simulink model "Scenario_3"  (R2020b)
settings: Solver=ode1  StartTime=0.0  StopTime=10.0  RelTol=1e-3
InitFcn:
  | Scenario_3_parameters;
values from neighbouring files (symbols this model uses):
  c0 = c0_zeb    (= 6.57988e-09)    [Scenario_17_parameters.m]    (also in Scenario_1_parameters.m = 6.37282e-09; Scenario_2_parameters.m = 6.37282e-09; Scenario_3_parameters.m)
  c0_hawk = 6.37282e-09    [Scenario_17_parameters.m]    (also in Scenario_1_parameters.m; Scenario_2_parameters.m; Scenario_3_parameters.m)
  c1 = c1_zeb    (= 9.15905e-09)    [Scenario_17_parameters.m]    (also in Scenario_1_parameters.m = 8.76156e-09; Scenario_2_parameters.m = 8.76156e-09; Scenario_3_parameters.m)
  c1_hawk = 8.76156e-09    [Scenario_17_parameters.m]    (also in Scenario_1_parameters.m; Scenario_2_parameters.m; Scenario_3_parameters.m)
  fg = 50    [Scenario_17_parameters.m]    (also in Scenario_1_parameters.m; Scenario_2_parameters.m; Scenario_3_parameters.m)
  G10gen = 0.85    [Scenario_3_parameters.m]
  G12gen = 0.85    [Scenario_3_parameters.m]
  G1gen = 0.50    (= 0.5)    [Scenario_17_parameters.m]    (also in Scenario_1_parameters.m = 0.2; Scenario_2_parameters.m = 0.1245; Scenario_3_parameters.m = 0.45)
  G2gen = 0.30    (= 0.3)    [Scenario_1_parameters.m]    (also in Scenario_2_parameters.m; Scenario_3_parameters.m = 0.4)
  G3gen = 0.25    [Scenario_1_parameters.m]    (also in Scenario_2_parameters.m = 0.2; Scenario_3_parameters.m = 0.6)
  G4gen = 0.95    [Scenario_3_parameters.m]
  G5gen = 0.75    [Scenario_17_parameters.m]    (also in Scenario_1_parameters.m = 0.22; Scenario_2_parameters.m = 0.2; Scenario_3_parameters.m = 0.7)
  G6gen = 0.90    (= 0.9)    [Scenario_17_parameters.m]    (also in Scenario_1_parameters.m = 0.41; Scenario_2_parameters.m = 0.2078; Scenario_3_parameters.m = 0.95)
  G7gen = 0.60    (= 0.6)    [Scenario_17_parameters.m]    (also in Scenario_1_parameters.m = 0.52; Scenario_2_parameters.m = 0.518; Scenario_3_parameters.m = 0.5)
  G8gen = 0.55    [Scenario_17_parameters.m]    (also in Scenario_3_parameters.m = 0.65)
  G9gen = 0.85    [Scenario_17_parameters.m]    (also in Scenario_3_parameters.m = 0.75)
  Ihvpk = Ihv*sqrt(2)    [Scenario_17_parameters.m]    (also in Scenario_1_parameters.m; Scenario_2_parameters.m; Scenario_3_parameters.m)
  l0 = l0_zeb    (= 0.00368)    [Scenario_17_parameters.m]    (also in Scenario_1_parameters.m = 0.00373; Scenario_2_parameters.m = 0.00373; Scenario_3_parameters.m)
  l0_hawk = 0.00373    [Scenario_17_parameters.m]    (also in Scenario_1_parameters.m; Scenario_2_parameters.m; Scenario_3_parameters.m)
  l1 = l1_zeb    (= 0.00128)    [Scenario_17_parameters.m]    (also in Scenario_1_parameters.m = 0.00133; Scenario_2_parameters.m = 0.00133; Scenario_3_parameters.m)
  L10dem = 0.10    (= 0.1)    [Scenario_3_parameters.m]
  L12dem = 0.025    [Scenario_17_parameters.m]    (also in Scenario_3_parameters.m = 0.005)
  L13dem = 0.005    [Scenario_3_parameters.m]
  l1_hawk = 0.00133    [Scenario_17_parameters.m]    (also in Scenario_1_parameters.m; Scenario_2_parameters.m; Scenario_3_parameters.m)
  L1dem = 0.25    [Scenario_17_parameters.m]    (also in Scenario_3_parameters.m = 0.1)
  L3dem = 0.30    (= 0.3)    [Scenario_17_parameters.m]    (also in Scenario_1_parameters.m = 0.1; Scenario_2_parameters.m = 0.1; Scenario_3_parameters.m = 0.2)
  L6dem = 0.15    [Scenario_1_parameters.m]    (also in Scenario_2_parameters.m; Scenario_3_parameters.m = 0.1)
  L7dem = 0.10    (= 0.1)    [Scenario_1_parameters.m]    (also in Scenario_2_parameters.m; Scenario_3_parameters.m = 0.15)
  L9dem = 0.15    [Scenario_17_parameters.m]    (also in Scenario_3_parameters.m)
  Pr = Sr*PF    (= 1900000000)    [Scenario_17_parameters.m]    (also in Scenario_1_parameters.m = 550050000; Scenario_2_parameters.m = 550050000; Scenario_3_parameters.m = 11640000000)
  Qr = sqrt(Sr^2 - Pr^2)    [Scenario_17_parameters.m]    (also in Scenario_1_parameters.m; Scenario_2_parameters.m; Scenario_3_parameters.m)
  r0 = r0_zeb    (= 0.39362)    [Scenario_17_parameters.m]    (also in Scenario_1_parameters.m = 0.44587; Scenario_2_parameters.m = 0.44587; Scenario_3_parameters.m)
  r0_hawk = 0.44587    [Scenario_17_parameters.m]    (also in Scenario_1_parameters.m; Scenario_2_parameters.m; Scenario_3_parameters.m)
  r1 = r1_zeb    (= 0.06862)    [Scenario_17_parameters.m]    (also in Scenario_1_parameters.m = 0.12087; Scenario_2_parameters.m = 0.12087; Scenario_3_parameters.m)
  r1_hawk = 0.12087    [Scenario_17_parameters.m]    (also in Scenario_1_parameters.m; Scenario_2_parameters.m; Scenario_3_parameters.m)
  Rtpu = Xtpu/40    (= 0.0025)    [Scenario_17_parameters.m]    (also in Scenario_1_parameters.m = 0.00375; Scenario_2_parameters.m = 0.00375; Scenario_3_parameters.m = 0.00375)
  S10non = 500e6    (= 500000000)    [Scenario_3_parameters.m]
  S12non = 1500e6    (= 1500000000)    [Scenario_3_parameters.m]
  S1non = 700e6    (= 700000000)    [Scenario_17_parameters.m]    (also in Scenario_1_parameters.m = 400000000; Scenario_2_parameters.m = 400000000; Scenario_3_parameters.m = 1000000000)
  S2non = 300e6    (= 300000000)    [Scenario_1_parameters.m]    (also in Scenario_2_parameters.m; Scenario_3_parameters.m = 3000000000)
  S3non = 200e6    (= 200000000)    [Scenario_1_parameters.m]    (also in Scenario_2_parameters.m; Scenario_3_parameters.m = 1000000000)
  S4non = 2000e6    (= 2000000000)    [Scenario_3_parameters.m]
  S5non = 400e6    (= 400000000)    [Scenario_17_parameters.m]    (also in Scenario_1_parameters.m = 500000000; Scenario_2_parameters.m = 500000000; Scenario_3_parameters.m = 2000000000)
  S6non = 150e6    (= 150000000)    [Scenario_17_parameters.m]    (also in Scenario_1_parameters.m = 400000000; Scenario_2_parameters.m = 400000000; Scenario_3_parameters.m = 3000000000)
  S7non = 1000e6    (= 1000000000)    [Scenario_17_parameters.m]    (also in Scenario_1_parameters.m = 200000000; Scenario_2_parameters.m = 200000000; Scenario_3_parameters.m = 4000000000)
  S8non = 600e6    (= 600000000)    [Scenario_17_parameters.m]    (also in Scenario_3_parameters.m = 2000000000)
  S9non = 200e6    (= 200000000)    [Scenario_17_parameters.m]    (also in Scenario_3_parameters.m = 1500000000)
  tonvsc = 0.01    [Scenario_17_parameters.m]    (also in Scenario_1_parameters.m = 0.02; Scenario_2_parameters.m; Scenario_3_parameters.m = 0.05)
  Ts = 100e-6    (= 0.0001)    [Scenario_17_parameters.m]    (also in Scenario_1_parameters.m; Scenario_2_parameters.m; Scenario_3_parameters.m = 5e-05)
  Vhv = 220e3    (= 220000)    [Scenario_17_parameters.m]    (also in Scenario_1_parameters.m; Scenario_2_parameters.m; Scenario_3_parameters.m)
  Vmv = 22e3    (= 22000)    [Scenario_17_parameters.m]    (also in Scenario_1_parameters.m; Scenario_2_parameters.m; Scenario_3_parameters.m)
  wc1 = wsw1/10    (= 848.230016469)    [Scenario_17_parameters.m]    (also in Scenario_1_parameters.m; Scenario_2_parameters.m; Scenario_3_parameters.m)
  wdc1 = wc1/10    (= 84.8230016469)    [Scenario_17_parameters.m]    (also in Scenario_1_parameters.m; Scenario_2_parameters.m; Scenario_3_parameters.m)
  wpq1 = wc1/10    (= 84.8230016469)    [Scenario_17_parameters.m]    (also in Scenario_1_parameters.m; Scenario_2_parameters.m; Scenario_3_parameters.m)
  wsw1 = ksw1*2*pi*fg    (= 8482.30016469)    [Scenario_17_parameters.m]    (also in Scenario_1_parameters.m; Scenario_2_parameters.m; Scenario_3_parameters.m)
  Xtpu = 0.10    (= 0.1)    [Scenario_17_parameters.m]    (also in Scenario_1_parameters.m = 0.15; Scenario_2_parameters.m = 0.15; Scenario_3_parameters.m = 0.15)
undefined symbols (not defined in the file or in its folder): D11, Delta, Kf, r, theta0
libraries: powerlib x426, simulink_extras x305, powerlib_meascontrol x139, pid_lib x109, eeGeneralControl x72, simulink x60, eeTransforms x54, spsFirstOrderFilterLib x36, eePwmGeneratorTwoLevel x9
(part 10 of 36)

== system Scenario_3/G4/VSC/VSC Model/EMT AVG ==
  Ref : Inport
  Controlled Voltage Source3 : powerlib/Electrical Sources/Controlled Voltage Source  Initialize=off  Source_Type=AC  Amplitude=Vhvpk  Phase=0  Frequency=fg  Measurements=None
  Controlled Voltage Source4 : powerlib/Electrical Sources/Controlled Voltage Source  Initialize=off  Source_Type=AC  Amplitude=Vhvpk  Phase=-2*pi/3  Frequency=fg  Measurements=None
  Controlled Voltage Source5 : powerlib/Electrical Sources/Controlled Voltage Source  Initialize=off  Source_Type=AC  Amplitude=Vhvpk  Phase=-4*pi/3  Frequency=fg  Measurements=None
  Demux1 : Demux  Outputs=3
  Ground : powerlib/Elements/Ground  LConnTagsString=a
  Ground4 : powerlib/Elements/Ground  LConnTagsString=a
  Ground5 : powerlib/Elements/Ground  LConnTagsString=a
  A : PMIOPort  Side=Left
  B : PMIOPort  Port=2  Side=Left
  C : PMIOPort  Port=3  Side=Left
  wires:
  Ref/1 -> Demux1/1
  Demux1/1 -> Controlled Voltage Source3/1
  Demux1/2 -> Controlled Voltage Source4/1
  Demux1/3 -> Controlled Voltage Source5/1
  connections:
  Controlled Voltage Source3/RConn1 -- A/RConn1
  Controlled Voltage Source4/RConn1 -- B/RConn1
  Controlled Voltage Source5/RConn1 -- C/RConn1
  Ground/LConn1 -- Controlled Voltage Source3/LConn1
  Ground4/LConn1 -- Controlled Voltage Source4/LConn1
  Ground5/LConn1 -- Controlled Voltage Source5/LConn1

== system Scenario_3/G4/VSC/VSC Model/EMT SW ==
  Ref : Inport
  DC Voltage Source : powerlib/Electrical Sources/DC Voltage Source  Amplitude=Vdc  Measurements=None
  Universal Bridge : powerlib/Power Electronics/Universal Bridge  Arms=3  SnubberResistance=1e6  SnubberCapacitance=inf  Device=IGBT / Diodes  Ron=1e-4  Lon=0  ForwardVoltages="[  0  0  ]"  ForwardVoltage=0  GTOparameters=[ 10e-6 , 20e-6 ]  IGBTparameters=[ 1e-6 , 2e-6 ]  Measurements=None  Measurements_2=None  converterType=Rectifier
  A : PMIOPort  Side=Left
  B : PMIOPort  Port=2  Side=Left
  C : PMIOPort  Port=3  Side=Left
  wires:
  Ref/1 -> Universal Bridge/1
  connections:
  Universal Bridge/LConn2 -- B/RConn1
  Universal Bridge/LConn1 -- A/RConn1
  Universal Bridge/LConn3 -- C/RConn1
  Universal Bridge/RConn1 -- DC Voltage Source/RConn1
  Universal Bridge/RConn2 -- DC Voltage Source/LConn1

== system Scenario_3/G4/VSC/VSC Model/Phasor ==
  Ref : Inport
  Controlled Current Source : powerlib/Electrical Sources/Controlled Current Source  Initialize=off  Source_Type=AC  Amplitude=0  Phase=0  Frequency=0  Measurements=None
  Controlled Current Source1 : powerlib/Electrical Sources/Controlled Current Source  Initialize=off  Source_Type=AC  Amplitude=0  Phase=0  Frequency=0  Measurements=None
  Controlled Current Source2 : powerlib/Electrical Sources/Controlled Current Source  Initialize=off  Source_Type=AC  Amplitude=0  Phase=0  Frequency=0  Measurements=None
  Demux1 : Demux  Outputs=3
  Ground{1..3,5} (4 alike) : powerlib/Elements/Ground  LConnTagsString=a
  Three-Phase Series RLC Branch : powerlib/Elements/Three-Phase Series RLC Branch  LConnTagsString=A|B|C  RConnTagsString=A|B|C  BranchType=R  Resistance=1e7  Inductance=1e-3  Capacitance=1e-6  Measurements=None
  A : PMIOPort  Side=Left
  B : PMIOPort  Port=2  Side=Left
  C : PMIOPort  Port=3  Side=Left
  wires:
  [c] -> Controlled Current Source2/1
  [b] -> Controlled Current Source1/1
  [a] -> Controlled Current Source/1
  Demux1/3 -> [c]
  Demux1/2 -> [b]
  Demux1/1 -> [a]
  Ref/1 -> Demux1/1
  connections:
  Controlled Current Source/RConn1 -- Ground1/LConn1
  Controlled Current Source1/RConn1 -- Ground2/LConn1
  Controlled Current Source2/RConn1 -- Ground3/LConn1
  A/RConn1 -- Controlled Current Source/LConn1 -- Three-Phase Series RLC Branch/LConn1
  C/RConn1 -- Controlled Current Source2/LConn1 -- Three-Phase Series RLC Branch/LConn3
  Ground5/LConn1 -- Three-Phase Series RLC Branch/RConn2 -- Three-Phase Series RLC Branch/RConn1 -- Three-Phase Series RLC Branch/RConn3
  Controlled Current Source1/LConn1 -- Three-Phase Series RLC Branch/LConn2 -- B/RConn1

== system Scenario_3/G6/VSC/VSC Control/Control loops ==
  note: 1) Add Subsystem or Model blocks as valid variant choices.
      | 2) You cannot connect blocks at this level. At simulation, connectivity is automatically
      | determined, based on the active variant and port name matching.
  Pset : Inport
  Qset : Inport  Port=2
  vqd+- : Inport  Port=3
  iqd+- : Inport  Port=4
  freq : Inport  Port=5
  Block : Inport  Port=6
  Phasor I 1st : Subsystem  VariantControl=Phasor_I_1st
  Phasor I ref : Subsystem  VariantControl=Phasor_I_ref
  Phasor PQ 1st : Subsystem  VariantControl=Phasor_PQ
  "SW, EMT AVG, Phasor Quasi-EMT" : Subsystem  VariantControl=EMT_and_QEMT
  vqd+-ref : Outport
  iqd+-ref : Outport  Port=2
  m : Outport  Port=3

== system Scenario_3/G6/VSC/VSC Control/Measurements ==
  note: 1) Add Subsystem or Model blocks as valid variant choices.
      | 2) You cannot connect blocks at this level. At simulation, connectivity is automatically
      | determined, based on the active variant and port name matching.
  Vabc : Inport
  Iabc : Inport  Port=2
  EMT : Subsystem  VariantControl=EMT
  Phasor : Subsystem  VariantControl=Phasor
  vqd+- : Outport
  iqd+- : Outport  Port=2
  freq : Outport  Port=3
  theta : Outport  Port=4
  PQabc : Outport  Port=5

== system Scenario_3/G6/VSC/VSC Control/Modulation ==
  note: 1) Add Subsystem or Model blocks as valid variant choices.
      | 2) You cannot connect blocks at this level. At simulation, connectivity is automatically
      | determined, based on the active variant and port name matching.
  vqd+- : Inport
  vqd+-* : Inport  Port=2
  iqd+-* : Inport  Port=3
  theta : Inport  Port=4
  EMT AVG : Subsystem  VariantControl=EMT_AVG
  EMT Switching : Subsystem  VariantControl=EMT_SW
  Phasor I and Phasor PQ : Subsystem  VariantControl=Phasor_I_and_PQ
  Phasor Quasi-EMT : Subsystem  VariantControl=Phasor_QEMT
  Ref : Outport

== system Scenario_3/G6/VSC/VSC Model/EMT AVG ==
  Ref : Inport
  Controlled Voltage Source3 : powerlib/Electrical Sources/Controlled Voltage Source  Initialize=off  Source_Type=AC  Amplitude=Vhvpk  Phase=0  Frequency=fg  Measurements=None
  Controlled Voltage Source4 : powerlib/Electrical Sources/Controlled Voltage Source  Initialize=off  Source_Type=AC  Amplitude=Vhvpk  Phase=-2*pi/3  Frequency=fg  Measurements=None
  Controlled Voltage Source5 : powerlib/Electrical Sources/Controlled Voltage Source  Initialize=off  Source_Type=AC  Amplitude=Vhvpk  Phase=-4*pi/3  Frequency=fg  Measurements=None
  Demux1 : Demux  Outputs=3
  Ground : powerlib/Elements/Ground  LConnTagsString=a
  Ground4 : powerlib/Elements/Ground  LConnTagsString=a
  Ground5 : powerlib/Elements/Ground  LConnTagsString=a
  A : PMIOPort  Side=Left
  B : PMIOPort  Port=2  Side=Left
  C : PMIOPort  Port=3  Side=Left
  wires:
  Ref/1 -> Demux1/1
  Demux1/1 -> Controlled Voltage Source3/1
  Demux1/2 -> Controlled Voltage Source4/1
  Demux1/3 -> Controlled Voltage Source5/1
  connections:
  Controlled Voltage Source3/RConn1 -- A/RConn1
  Controlled Voltage Source4/RConn1 -- B/RConn1
  Controlled Voltage Source5/RConn1 -- C/RConn1
  Ground/LConn1 -- Controlled Voltage Source3/LConn1
  Ground4/LConn1 -- Controlled Voltage Source4/LConn1
  Ground5/LConn1 -- Controlled Voltage Source5/LConn1

== system Scenario_3/G6/VSC/VSC Model/EMT SW ==
  Ref : Inport
  DC Voltage Source : powerlib/Electrical Sources/DC Voltage Source  Amplitude=Vdc  Measurements=None
  Universal Bridge : powerlib/Power Electronics/Universal Bridge  Arms=3  SnubberResistance=1e6  SnubberCapacitance=inf  Device=IGBT / Diodes  Ron=1e-4  Lon=0  ForwardVoltages="[  0  0  ]"  ForwardVoltage=0  GTOparameters=[ 10e-6 , 20e-6 ]  IGBTparameters=[ 1e-6 , 2e-6 ]  Measurements=None  Measurements_2=None  converterType=Rectifier
  A : PMIOPort  Side=Left
  B : PMIOPort  Port=2  Side=Left
  C : PMIOPort  Port=3  Side=Left
  wires:
  Ref/1 -> Universal Bridge/1
  connections:
  Universal Bridge/LConn2 -- B/RConn1
  Universal Bridge/LConn1 -- A/RConn1
  Universal Bridge/LConn3 -- C/RConn1
  Universal Bridge/RConn1 -- DC Voltage Source/RConn1
  Universal Bridge/RConn2 -- DC Voltage Source/LConn1

== system Scenario_3/G6/VSC/VSC Model/Phasor ==
  Ref : Inport
  Controlled Current Source : powerlib/Electrical Sources/Controlled Current Source  Initialize=off  Source_Type=AC  Amplitude=0  Phase=0  Frequency=0  Measurements=None
  Controlled Current Source1 : powerlib/Electrical Sources/Controlled Current Source  Initialize=off  Source_Type=AC  Amplitude=0  Phase=0  Frequency=0  Measurements=None
  Controlled Current Source2 : powerlib/Electrical Sources/Controlled Current Source  Initialize=off  Source_Type=AC  Amplitude=0  Phase=0  Frequency=0  Measurements=None
  Demux1 : Demux  Outputs=3
  Ground{1..3,5} (4 alike) : powerlib/Elements/Ground  LConnTagsString=a
  Three-Phase Series RLC Branch : powerlib/Elements/Three-Phase Series RLC Branch  LConnTagsString=A|B|C  RConnTagsString=A|B|C  BranchType=R  Resistance=1e7  Inductance=1e-3  Capacitance=1e-6  Measurements=None
  A : PMIOPort  Side=Left
  B : PMIOPort  Port=2  Side=Left
  C : PMIOPort  Port=3  Side=Left
  wires:
  [c] -> Controlled Current Source2/1
  [b] -> Controlled Current Source1/1
  [a] -> Controlled Current Source/1
  Demux1/3 -> [c]
  Demux1/2 -> [b]
  Demux1/1 -> [a]
  Ref/1 -> Demux1/1
  connections:
  Controlled Current Source/RConn1 -- Ground1/LConn1
  Controlled Current Source1/RConn1 -- Ground2/LConn1
  Controlled Current Source2/RConn1 -- Ground3/LConn1
  A/RConn1 -- Controlled Current Source/LConn1 -- Three-Phase Series RLC Branch/LConn1
  C/RConn1 -- Controlled Current Source2/LConn1 -- Three-Phase Series RLC Branch/LConn3
  Ground5/LConn1 -- Three-Phase Series RLC Branch/RConn2 -- Three-Phase Series RLC Branch/RConn1 -- Three-Phase Series RLC Branch/RConn3
  Controlled Current Source1/LConn1 -- Three-Phase Series RLC Branch/LConn2 -- B/RConn1

== system Scenario_3/G7/VSC/VSC Control/Control loops ==
  note: 1) Add Subsystem or Model blocks as valid variant choices.
      | 2) You cannot connect blocks at this level. At simulation, connectivity is automatically
      | determined, based on the active variant and port name matching.
  Pset : Inport
  Qset : Inport  Port=2
  vqd+- : Inport  Port=3
  iqd+- : Inport  Port=4
  freq : Inport  Port=5
  Block : Inport  Port=6
  Phasor I 1st : Subsystem  VariantControl=Phasor_I_1st
  Phasor I ref : Subsystem  VariantControl=Phasor_I_ref
  Phasor PQ 1st : Subsystem  VariantControl=Phasor_PQ
  "SW, EMT AVG, Phasor Quasi-EMT" : Subsystem  VariantControl=EMT_and_QEMT
  vqd+-ref : Outport
  iqd+-ref : Outport  Port=2
  m : Outport  Port=3

== system Scenario_3/G7/VSC/VSC Control/Measurements ==
  note: 1) Add Subsystem or Model blocks as valid variant choices.
      | 2) You cannot connect blocks at this level. At simulation, connectivity is automatically
      | determined, based on the active variant and port name matching.
  Vabc : Inport
  Iabc : Inport  Port=2
  EMT : Subsystem  VariantControl=EMT
  Phasor : Subsystem  VariantControl=Phasor
  vqd+- : Outport
  iqd+- : Outport  Port=2
  freq : Outport  Port=3
  theta : Outport  Port=4
  PQabc : Outport  Port=5

== system Scenario_3/G7/VSC/VSC Control/Modulation ==
  note: 1) Add Subsystem or Model blocks as valid variant choices.
      | 2) You cannot connect blocks at this level. At simulation, connectivity is automatically
      | determined, based on the active variant and port name matching.
  vqd+- : Inport
  vqd+-* : Inport  Port=2
  iqd+-* : Inport  Port=3
  theta : Inport  Port=4
  EMT AVG : Subsystem  VariantControl=EMT_AVG
  EMT Switching : Subsystem  VariantControl=EMT_SW
  Phasor I and Phasor PQ : Subsystem  VariantControl=Phasor_I_and_PQ
  Phasor Quasi-EMT : Subsystem  VariantControl=Phasor_QEMT
  Ref : Outport

== system Scenario_3/G7/VSC/VSC Model/EMT AVG ==
  Ref : Inport
  Controlled Voltage Source3 : powerlib/Electrical Sources/Controlled Voltage Source  Initialize=off  Source_Type=AC  Amplitude=Vhvpk  Phase=0  Frequency=fg  Measurements=None
  Controlled Voltage Source4 : powerlib/Electrical Sources/Controlled Voltage Source  Initialize=off  Source_Type=AC  Amplitude=Vhvpk  Phase=-2*pi/3  Frequency=fg  Measurements=None
  Controlled Voltage Source5 : powerlib/Electrical Sources/Controlled Voltage Source  Initialize=off  Source_Type=AC  Amplitude=Vhvpk  Phase=-4*pi/3  Frequency=fg  Measurements=None
  Demux1 : Demux  Outputs=3
  Ground : powerlib/Elements/Ground  LConnTagsString=a
  Ground4 : powerlib/Elements/Ground  LConnTagsString=a
  Ground5 : powerlib/Elements/Ground  LConnTagsString=a
  A : PMIOPort  Side=Left
  B : PMIOPort  Port=2  Side=Left
  C : PMIOPort  Port=3  Side=Left
  wires:
  Ref/1 -> Demux1/1
  Demux1/1 -> Controlled Voltage Source3/1
  Demux1/2 -> Controlled Voltage Source4/1
  Demux1/3 -> Controlled Voltage Source5/1
  connections:
  Controlled Voltage Source3/RConn1 -- A/RConn1
  Controlled Voltage Source4/RConn1 -- B/RConn1
  Controlled Voltage Source5/RConn1 -- C/RConn1
  Ground/LConn1 -- Controlled Voltage Source3/LConn1
  Ground4/LConn1 -- Controlled Voltage Source4/LConn1
  Ground5/LConn1 -- Controlled Voltage Source5/LConn1

== system Scenario_3/G7/VSC/VSC Model/EMT SW ==
  Ref : Inport
  DC Voltage Source : powerlib/Electrical Sources/DC Voltage Source  Amplitude=Vdc  Measurements=None
  Universal Bridge : powerlib/Power Electronics/Universal Bridge  Arms=3  SnubberResistance=1e6  SnubberCapacitance=inf  Device=IGBT / Diodes  Ron=1e-4  Lon=0  ForwardVoltages="[  0  0  ]"  ForwardVoltage=0  GTOparameters=[ 10e-6 , 20e-6 ]  IGBTparameters=[ 1e-6 , 2e-6 ]  Measurements=None  Measurements_2=None  converterType=Rectifier
  A : PMIOPort  Side=Left
  B : PMIOPort  Port=2  Side=Left
  C : PMIOPort  Port=3  Side=Left
  wires:
  Ref/1 -> Universal Bridge/1
  connections:
  Universal Bridge/LConn2 -- B/RConn1
  Universal Bridge/LConn1 -- A/RConn1
  Universal Bridge/LConn3 -- C/RConn1
  Universal Bridge/RConn1 -- DC Voltage Source/RConn1
  Universal Bridge/RConn2 -- DC Voltage Source/LConn1

== system Scenario_3/G7/VSC/VSC Model/Phasor ==
  Ref : Inport
  Controlled Current Source : powerlib/Electrical Sources/Controlled Current Source  Initialize=off  Source_Type=AC  Amplitude=0  Phase=0  Frequency=0  Measurements=None
  Controlled Current Source1 : powerlib/Electrical Sources/Controlled Current Source  Initialize=off  Source_Type=AC  Amplitude=0  Phase=0  Frequency=0  Measurements=None
  Controlled Current Source2 : powerlib/Electrical Sources/Controlled Current Source  Initialize=off  Source_Type=AC  Amplitude=0  Phase=0  Frequency=0  Measurements=None
  Demux1 : Demux  Outputs=3
  Ground{1..3,5} (4 alike) : powerlib/Elements/Ground  LConnTagsString=a
  Three-Phase Series RLC Branch : powerlib/Elements/Three-Phase Series RLC Branch  LConnTagsString=A|B|C  RConnTagsString=A|B|C  BranchType=R  Resistance=1e7  Inductance=1e-3  Capacitance=1e-6  Measurements=None
  A : PMIOPort  Side=Left
  B : PMIOPort  Port=2  Side=Left
  C : PMIOPort  Port=3  Side=Left
  wires:
  [c] -> Controlled Current Source2/1
  [b] -> Controlled Current Source1/1
  [a] -> Controlled Current Source/1
  Demux1/3 -> [c]
  Demux1/2 -> [b]
  Demux1/1 -> [a]
  Ref/1 -> Demux1/1
  connections:
  Controlled Current Source/RConn1 -- Ground1/LConn1
  Controlled Current Source1/RConn1 -- Ground2/LConn1
  Controlled Current Source2/RConn1 -- Ground3/LConn1
  A/RConn1 -- Controlled Current Source/LConn1 -- Three-Phase Series RLC Branch/LConn1
  C/RConn1 -- Controlled Current Source2/LConn1 -- Three-Phase Series RLC Branch/LConn3
  Ground5/LConn1 -- Three-Phase Series RLC Branch/RConn2 -- Three-Phase Series RLC Branch/RConn1 -- Three-Phase Series RLC Branch/RConn3
  Controlled Current Source1/LConn1 -- Three-Phase Series RLC Branch/LConn2 -- B/RConn1

== system Scenario_3/G9/VSC/VSC Control/Control loops ==
  note: 1) Add Subsystem or Model blocks as valid variant choices.
      | 2) You cannot connect blocks at this level. At simulation, connectivity is automatically
      | determined, based on the active variant and port name matching.
  Pset : Inport
  Qset : Inport  Port=2
  vqd+- : Inport  Port=3
  iqd+- : Inport  Port=4
  freq : Inport  Port=5
  Block : Inport  Port=6
  Phasor I 1st : Subsystem  VariantControl=Phasor_I_1st
  Phasor I ref : Subsystem  VariantControl=Phasor_I_ref
  Phasor PQ 1st : Subsystem  VariantControl=Phasor_PQ
  "SW, EMT AVG, Phasor Quasi-EMT" : Subsystem  VariantControl=EMT_and_QEMT
  vqd+-ref : Outport
  iqd+-ref : Outport  Port=2
  m : Outport  Port=3

== system Scenario_3/G9/VSC/VSC Control/Measurements ==
  note: 1) Add Subsystem or Model blocks as valid variant choices.
      | 2) You cannot connect blocks at this level. At simulation, connectivity is automatically
      | determined, based on the active variant and port name matching.
  Vabc : Inport
  Iabc : Inport  Port=2
  EMT : Subsystem  VariantControl=EMT
  Phasor : Subsystem  VariantControl=Phasor
  vqd+- : Outport
  iqd+- : Outport  Port=2
  freq : Outport  Port=3
  theta : Outport  Port=4
  PQabc : Outport  Port=5

== system Scenario_3/G9/VSC/VSC Control/Modulation ==
  note: 1) Add Subsystem or Model blocks as valid variant choices.
      | 2) You cannot connect blocks at this level. At simulation, connectivity is automatically
      | determined, based on the active variant and port name matching.
  vqd+- : Inport
  vqd+-* : Inport  Port=2
  iqd+-* : Inport  Port=3
  theta : Inport  Port=4
  EMT AVG : Subsystem  VariantControl=EMT_AVG
  EMT Switching : Subsystem  VariantControl=EMT_SW
  Phasor I and Phasor PQ : Subsystem  VariantControl=Phasor_I_and_PQ
  Phasor Quasi-EMT : Subsystem  VariantControl=Phasor_QEMT
  Ref : Outport

== system Scenario_3/G9/VSC/VSC Model/EMT AVG ==
  Ref : Inport
  Controlled Voltage Source3 : powerlib/Electrical Sources/Controlled Voltage Source  Initialize=off  Source_Type=AC  Amplitude=Vhvpk  Phase=0  Frequency=fg  Measurements=None
  Controlled Voltage Source4 : powerlib/Electrical Sources/Controlled Voltage Source  Initialize=off  Source_Type=AC  Amplitude=Vhvpk  Phase=-2*pi/3  Frequency=fg  Measurements=None
  Controlled Voltage Source5 : powerlib/Electrical Sources/Controlled Voltage Source  Initialize=off  Source_Type=AC  Amplitude=Vhvpk  Phase=-4*pi/3  Frequency=fg  Measurements=None
  Demux1 : Demux  Outputs=3
  Ground : powerlib/Elements/Ground  LConnTagsString=a
  Ground4 : powerlib/Elements/Ground  LConnTagsString=a
  Ground5 : powerlib/Elements/Ground  LConnTagsString=a
  A : PMIOPort  Side=Left
  B : PMIOPort  Port=2  Side=Left
  C : PMIOPort  Port=3  Side=Left
  wires:
  Ref/1 -> Demux1/1
  Demux1/1 -> Controlled Voltage Source3/1
  Demux1/2 -> Controlled Voltage Source4/1
  Demux1/3 -> Controlled Voltage Source5/1
  connections:
  Controlled Voltage Source3/RConn1 -- A/RConn1
  Controlled Voltage Source4/RConn1 -- B/RConn1
  Controlled Voltage Source5/RConn1 -- C/RConn1
  Ground/LConn1 -- Controlled Voltage Source3/LConn1
  Ground4/LConn1 -- Controlled Voltage Source4/LConn1
  Ground5/LConn1 -- Controlled Voltage Source5/LConn1

== system Scenario_3/G9/VSC/VSC Model/EMT SW ==
  Ref : Inport
  DC Voltage Source : powerlib/Electrical Sources/DC Voltage Source  Amplitude=Vdc  Measurements=None
  Universal Bridge : powerlib/Power Electronics/Universal Bridge  Arms=3  SnubberResistance=1e6  SnubberCapacitance=inf  Device=IGBT / Diodes  Ron=1e-4  Lon=0  ForwardVoltages="[  0  0  ]"  ForwardVoltage=0  GTOparameters=[ 10e-6 , 20e-6 ]  IGBTparameters=[ 1e-6 , 2e-6 ]  Measurements=None  Measurements_2=None  converterType=Rectifier
  A : PMIOPort  Side=Left
  B : PMIOPort  Port=2  Side=Left
  C : PMIOPort  Port=3  Side=Left
  wires:
  Ref/1 -> Universal Bridge/1
  connections:
  Universal Bridge/LConn2 -- B/RConn1
  Universal Bridge/LConn1 -- A/RConn1
  Universal Bridge/LConn3 -- C/RConn1
  Universal Bridge/RConn1 -- DC Voltage Source/RConn1
  Universal Bridge/RConn2 -- DC Voltage Source/LConn1

== system Scenario_3/G9/VSC/VSC Model/Phasor ==
  Ref : Inport
  Controlled Current Source : powerlib/Electrical Sources/Controlled Current Source  Initialize=off  Source_Type=AC  Amplitude=0  Phase=0  Frequency=0  Measurements=None
  Controlled Current Source1 : powerlib/Electrical Sources/Controlled Current Source  Initialize=off  Source_Type=AC  Amplitude=0  Phase=0  Frequency=0  Measurements=None
  Controlled Current Source2 : powerlib/Electrical Sources/Controlled Current Source  Initialize=off  Source_Type=AC  Amplitude=0  Phase=0  Frequency=0  Measurements=None
  Demux1 : Demux  Outputs=3
  Ground{1..3,5} (4 alike) : powerlib/Elements/Ground  LConnTagsString=a
  Three-Phase Series RLC Branch : powerlib/Elements/Three-Phase Series RLC Branch  LConnTagsString=A|B|C  RConnTagsString=A|B|C  BranchType=R  Resistance=1e7  Inductance=1e-3  Capacitance=1e-6  Measurements=None
  A : PMIOPort  Side=Left
  B : PMIOPort  Port=2  Side=Left
  C : PMIOPort  Port=3  Side=Left
  wires:
  [c] -> Controlled Current Source2/1
  [b] -> Controlled Current Source1/1
  [a] -> Controlled Current Source/1
  Demux1/3 -> [c]
  Demux1/2 -> [b]
  Demux1/1 -> [a]
  Ref/1 -> Demux1/1
  connections:
  Controlled Current Source/RConn1 -- Ground1/LConn1
  Controlled Current Source1/RConn1 -- Ground2/LConn1
  Controlled Current Source2/RConn1 -- Ground3/LConn1
  A/RConn1 -- Controlled Current Source/LConn1 -- Three-Phase Series RLC Branch/LConn1
  C/RConn1 -- Controlled Current Source2/LConn1 -- Three-Phase Series RLC Branch/LConn3
  Ground5/LConn1 -- Three-Phase Series RLC Branch/RConn2 -- Three-Phase Series RLC Branch/RConn1 -- Three-Phase Series RLC Branch/RConn3
  Controlled Current Source1/LConn1 -- Three-Phase Series RLC Branch/LConn2 -- B/RConn1

== system Scenario_3/HVDC interconnection/VSC1/VSC Control/Control loops ==
  note: 1) Add Subsystem or Model blocks as valid variant choices.
      | 2) You cannot connect blocks at this level. At simulation, connectivity is automatically
      | determined, based on the active variant and port name matching.
  Pset : Inport
  Qset : Inport  Port=2
  vqd+- : Inport  Port=3
  iqd+- : Inport  Port=4
  freq : Inport  Port=5
  Block : Inport  Port=6
  Phasor I 1st : Subsystem  VariantControl=Phasor_I_1st
  Phasor I ref : Subsystem  VariantControl=Phasor_I_ref
  Phasor PQ 1st : Subsystem  VariantControl=Phasor_PQ
  "SW, EMT AVG, Phasor Quasi-EMT" : Subsystem  VariantControl=EMT_and_QEMT
  vqd+-ref : Outport
  iqd+-ref : Outport  Port=2
  m : Outport  Port=3

== system Scenario_3/HVDC interconnection/VSC1/VSC Control/Measurements ==
  note: 1) Add Subsystem or Model blocks as valid variant choices.
      | 2) You cannot connect blocks at this level. At simulation, connectivity is automatically
      | determined, based on the active variant and port name matching.
  Vabc : Inport
  Iabc : Inport  Port=2
  EMT : Subsystem  VariantControl=EMT
  Phasor : Subsystem  VariantControl=Phasor
  vqd+- : Outport
  iqd+- : Outport  Port=2
  freq : Outport  Port=3
  theta : Outport  Port=4
  PQabc : Outport  Port=5

== system Scenario_3/HVDC interconnection/VSC1/VSC Control/Modulation ==
  note: 1) Add Subsystem or Model blocks as valid variant choices.
      | 2) You cannot connect blocks at this level. At simulation, connectivity is automatically
      | determined, based on the active variant and port name matching.
  vqd+- : Inport
  vqd+-* : Inport  Port=2
  iqd+-* : Inport  Port=3
  theta : Inport  Port=4
  EMT AVG : Subsystem  VariantControl=EMT_AVG
  EMT Switching : Subsystem  VariantControl=EMT_SW
  Phasor I and Phasor PQ : Subsystem  VariantControl=Phasor_I_and_PQ
  Phasor Quasi-EMT : Subsystem  VariantControl=Phasor_QEMT
  Ref : Outport

== system Scenario_3/HVDC interconnection/VSC1/VSC Model/EMT AVG ==
  Ref : Inport
  Controlled Voltage Source3 : powerlib/Electrical Sources/Controlled Voltage Source  Initialize=off  Source_Type=AC  Amplitude=Vhvpk  Phase=0  Frequency=fg  Measurements=None
  Controlled Voltage Source4 : powerlib/Electrical Sources/Controlled Voltage Source  Initialize=off  Source_Type=AC  Amplitude=Vhvpk  Phase=-2*pi/3  Frequency=fg  Measurements=None
  Controlled Voltage Source5 : powerlib/Electrical Sources/Controlled Voltage Source  Initialize=off  Source_Type=AC  Amplitude=Vhvpk  Phase=-4*pi/3  Frequency=fg  Measurements=None
  Demux1 : Demux  Outputs=3
  Ground : powerlib/Elements/Ground  LConnTagsString=a
  Ground4 : powerlib/Elements/Ground  LConnTagsString=a
  Ground5 : powerlib/Elements/Ground  LConnTagsString=a
  A : PMIOPort  Side=Left
  B : PMIOPort  Port=2  Side=Left
  C : PMIOPort  Port=3  Side=Left
  wires:
  Ref/1 -> Demux1/1
  Demux1/1 -> Controlled Voltage Source3/1
  Demux1/2 -> Controlled Voltage Source4/1
  Demux1/3 -> Controlled Voltage Source5/1
  connections:
  Controlled Voltage Source3/RConn1 -- A/RConn1
  Controlled Voltage Source4/RConn1 -- B/RConn1
  Controlled Voltage Source5/RConn1 -- C/RConn1
  Ground/LConn1 -- Controlled Voltage Source3/LConn1
  Ground4/LConn1 -- Controlled Voltage Source4/LConn1
  Ground5/LConn1 -- Controlled Voltage Source5/LConn1

== system Scenario_3/HVDC interconnection/VSC1/VSC Model/EMT SW ==
  Ref : Inport
  DC Voltage Source : powerlib/Electrical Sources/DC Voltage Source  Amplitude=Vdc  Measurements=None
  Universal Bridge : powerlib/Power Electronics/Universal Bridge  Arms=3  SnubberResistance=1e6  SnubberCapacitance=inf  Device=IGBT / Diodes  Ron=1e-4  Lon=0  ForwardVoltages="[  0  0  ]"  ForwardVoltage=0  GTOparameters=[ 10e-6 , 20e-6 ]  IGBTparameters=[ 1e-6 , 2e-6 ]  Measurements=None  Measurements_2=None  converterType=Rectifier
  A : PMIOPort  Side=Left
  B : PMIOPort  Port=2  Side=Left
  C : PMIOPort  Port=3  Side=Left
  wires:
  Ref/1 -> Universal Bridge/1
  connections:
  Universal Bridge/LConn2 -- B/RConn1
  Universal Bridge/LConn1 -- A/RConn1
  Universal Bridge/LConn3 -- C/RConn1
  Universal Bridge/RConn1 -- DC Voltage Source/RConn1
  Universal Bridge/RConn2 -- DC Voltage Source/LConn1

== system Scenario_3/HVDC interconnection/VSC1/VSC Model/Phasor ==
  Ref : Inport
  Controlled Current Source : powerlib/Electrical Sources/Controlled Current Source  Initialize=off  Source_Type=AC  Amplitude=0  Phase=0  Frequency=0  Measurements=None
  Controlled Current Source1 : powerlib/Electrical Sources/Controlled Current Source  Initialize=off  Source_Type=AC  Amplitude=0  Phase=0  Frequency=0  Measurements=None
  Controlled Current Source2 : powerlib/Electrical Sources/Controlled Current Source  Initialize=off  Source_Type=AC  Amplitude=0  Phase=0  Frequency=0  Measurements=None
  Demux1 : Demux  Outputs=3
  Ground{1..3,5} (4 alike) : powerlib/Elements/Ground  LConnTagsString=a
  Three-Phase Series RLC Branch : powerlib/Elements/Three-Phase Series RLC Branch  LConnTagsString=A|B|C  RConnTagsString=A|B|C  BranchType=R  Resistance=1e7  Inductance=1e-3  Capacitance=1e-6  Measurements=None
  A : PMIOPort  Side=Left
  B : PMIOPort  Port=2  Side=Left
  C : PMIOPort  Port=3  Side=Left
  wires:
  [c] -> Controlled Current Source2/1
  [b] -> Controlled Current Source1/1
  [a] -> Controlled Current Source/1
  Demux1/3 -> [c]
  Demux1/2 -> [b]
  Demux1/1 -> [a]
  Ref/1 -> Demux1/1
  connections:
  Controlled Current Source/RConn1 -- Ground1/LConn1
  Controlled Current Source1/RConn1 -- Ground2/LConn1
  Controlled Current Source2/RConn1 -- Ground3/LConn1
  A/RConn1 -- Controlled Current Source/LConn1 -- Three-Phase Series RLC Branch/LConn1
  C/RConn1 -- Controlled Current Source2/LConn1 -- Three-Phase Series RLC Branch/LConn3
  Ground5/LConn1 -- Three-Phase Series RLC Branch/RConn2 -- Three-Phase Series RLC Branch/RConn1 -- Three-Phase Series RLC Branch/RConn3
  Controlled Current Source1/LConn1 -- Three-Phase Series RLC Branch/LConn2 -- B/RConn1

== system Scenario_3/HVDC interconnection/VSC2/VSC Control/Control loops ==
  note: 1) Add Subsystem or Model blocks as valid variant choices.
      | 2) You cannot connect blocks at this level. At simulation, connectivity is automatically
      | determined, based on the active variant and port name matching.
  Pset : Inport
  Qset : Inport  Port=2
  vqd+- : Inport  Port=3
  iqd+- : Inport  Port=4
  freq : Inport  Port=5
  Block : Inport  Port=6
  Edc : Inport  Port=7
  Phasor I 1st : Subsystem  VariantControl=Phasor_I_1st
  Phasor I ref : Subsystem  VariantControl=Phasor_I_ref
  Phasor PQ 1st : Subsystem  VariantControl=Phasor_PQ
  "SW, EMT AVG, Phasor Quasi-EMT" : Subsystem  VariantControl=EMT_and_QEMT
  vqd+-ref : Outport
  iqd+-ref : Outport  Port=2
  m : Outport  Port=3

== system Scenario_3/HVDC interconnection/VSC2/VSC Control/Measurements ==
  note: 1) Add Subsystem or Model blocks as valid variant choices.
      | 2) You cannot connect blocks at this level. At simulation, connectivity is automatically
      | determined, based on the active variant and port name matching.
  Vabc : Inport
  Iabc : Inport  Port=2
  EMT : Subsystem  VariantControl=EMT
  Phasor : Subsystem  VariantControl=Phasor
  vqd+- : Outport
  iqd+- : Outport  Port=2
  freq : Outport  Port=3
  theta : Outport  Port=4
  PQabc : Outport  Port=5

== system Scenario_3/HVDC interconnection/VSC2/VSC Control/Modulation ==
  note: 1) Add Subsystem or Model blocks as valid variant choices.
      | 2) You cannot connect blocks at this level. At simulation, connectivity is automatically
      | determined, based on the active variant and port name matching.
  vqd+- : Inport
  vqd+-* : Inport  Port=2
  iqd+-* : Inport  Port=3
  theta : Inport  Port=4
  EMT AVG : Subsystem  VariantControl=EMT_AVG
  EMT Switching : Subsystem  VariantControl=EMT_SW
  Phasor I and Phasor PQ : Subsystem  VariantControl=Phasor_I_and_PQ
  Phasor Quasi-EMT : Subsystem  VariantControl=Phasor_QEMT
  Ref : Outport

== system Scenario_3/HVDC interconnection/VSC2/VSC Model/EMT AVG ==
  Ref : Inport
  Controlled Voltage Source3 : powerlib/Electrical Sources/Controlled Voltage Source  Initialize=off  Source_Type=AC  Amplitude=Vhvpk  Phase=0  Frequency=fg  Measurements=None
  Controlled Voltage Source4 : powerlib/Electrical Sources/Controlled Voltage Source  Initialize=off  Source_Type=AC  Amplitude=Vhvpk  Phase=-2*pi/3  Frequency=fg  Measurements=None
  Controlled Voltage Source5 : powerlib/Electrical Sources/Controlled Voltage Source  Initialize=off  Source_Type=AC  Amplitude=Vhvpk  Phase=-4*pi/3  Frequency=fg  Measurements=None
  Demux1 : Demux  Outputs=3
  Ground : powerlib/Elements/Ground  LConnTagsString=a
  Ground4 : powerlib/Elements/Ground  LConnTagsString=a
  Ground5 : powerlib/Elements/Ground  LConnTagsString=a
  A : PMIOPort  Side=Left
  B : PMIOPort  Port=2  Side=Left
  C : PMIOPort  Port=3  Side=Left
  wires:
  Ref/1 -> Demux1/1
  Demux1/1 -> Controlled Voltage Source3/1
  Demux1/2 -> Controlled Voltage Source4/1
  Demux1/3 -> Controlled Voltage Source5/1
  connections:
  Controlled Voltage Source3/RConn1 -- A/RConn1
  Controlled Voltage Source4/RConn1 -- B/RConn1
  Controlled Voltage Source5/RConn1 -- C/RConn1
  Ground/LConn1 -- Controlled Voltage Source3/LConn1
  Ground4/LConn1 -- Controlled Voltage Source4/LConn1
  Ground5/LConn1 -- Controlled Voltage Source5/LConn1

== system Scenario_3/HVDC interconnection/VSC2/VSC Model/EMT SW ==
  Ref : Inport
  DC Voltage Source : powerlib/Electrical Sources/DC Voltage Source  Amplitude=Vdc  Measurements=None
  Universal Bridge : powerlib/Power Electronics/Universal Bridge  Arms=3  SnubberResistance=1e6  SnubberCapacitance=inf  Device=IGBT / Diodes  Ron=1e-4  Lon=0  ForwardVoltages="[  0  0  ]"  ForwardVoltage=0  GTOparameters=[ 10e-6 , 20e-6 ]  IGBTparameters=[ 1e-6 , 2e-6 ]  Measurements=None  Measurements_2=None  converterType=Rectifier
  A : PMIOPort  Side=Left
  B : PMIOPort  Port=2  Side=Left
  C : PMIOPort  Port=3  Side=Left
  wires:
  Ref/1 -> Universal Bridge/1
  connections:
  Universal Bridge/LConn2 -- B/RConn1
  Universal Bridge/LConn1 -- A/RConn1
  Universal Bridge/LConn3 -- C/RConn1
  Universal Bridge/RConn1 -- DC Voltage Source/RConn1
  Universal Bridge/RConn2 -- DC Voltage Source/LConn1

== system Scenario_3/HVDC interconnection/VSC2/VSC Model/Phasor ==
  Ref : Inport
  Controlled Current Source : powerlib/Electrical Sources/Controlled Current Source  Initialize=off  Source_Type=AC  Amplitude=0  Phase=0  Frequency=0  Measurements=None
  Controlled Current Source1 : powerlib/Electrical Sources/Controlled Current Source  Initialize=off  Source_Type=AC  Amplitude=0  Phase=0  Frequency=0  Measurements=None
  Controlled Current Source2 : powerlib/Electrical Sources/Controlled Current Source  Initialize=off  Source_Type=AC  Amplitude=0  Phase=0  Frequency=0  Measurements=None
  Demux1 : Demux  Outputs=3
  Ground{1..3,5} (4 alike) : powerlib/Elements/Ground  LConnTagsString=a
  Three-Phase Series RLC Branch : powerlib/Elements/Three-Phase Series RLC Branch  LConnTagsString=A|B|C  RConnTagsString=A|B|C  BranchType=R  Resistance=1e7  Inductance=1e-3  Capacitance=1e-6  Measurements=None
  A : PMIOPort  Side=Left
  B : PMIOPort  Port=2  Side=Left
  C : PMIOPort  Port=3  Side=Left
  wires:
  [c] -> Controlled Current Source2/1
  [b] -> Controlled Current Source1/1
  [a] -> Controlled Current Source/1
  Demux1/3 -> [c]
  Demux1/2 -> [b]
  Demux1/1 -> [a]
  Ref/1 -> Demux1/1
  connections:
  Controlled Current Source/RConn1 -- Ground1/LConn1
  Controlled Current Source1/RConn1 -- Ground2/LConn1
  Controlled Current Source2/RConn1 -- Ground3/LConn1
  A/RConn1 -- Controlled Current Source/LConn1 -- Three-Phase Series RLC Branch/LConn1
  C/RConn1 -- Controlled Current Source2/LConn1 -- Three-Phase Series RLC Branch/LConn3
  Ground5/LConn1 -- Three-Phase Series RLC Branch/RConn2 -- Three-Phase Series RLC Branch/RConn1 -- Three-Phase Series RLC Branch/RConn3
  Controlled Current Source1/LConn1 -- Three-Phase Series RLC Branch/LConn2 -- B/RConn1

== system Scenario_3/G1/VSC/VSC Control/Control loops/Phasor I 1st ==
  Pset : Inport
  Qset : Inport  Port=2
  vqd+- : Inport  Port=3
  iqd+- : Inport  Port=4
  freq : Inport  Port=5
  Block : Inport  Port=6
  Inner-loop : Subsystem
  Mux : Mux
  Outer-loop : Subsystem
      settings: PortSchema="{\"entries\":[{\"content\":{\"sides\":[{\"content\":{\"connectorIds\":[\"In1\",\"In2\",\"In3\",\"In4\",\"In5\"]},\"type\":\"ConnectorPlacement.EquallySpacedRectSide\",\"uuid\":\"9a334ab0-c6a2-41fb-a6ec-750715335523\"},{\"content\":{\"connectorIds\":[\"Out1\",\"Out2\",\"Out3\",\"Out4\",\"Out5\"],\"side\":\"RIGHT\"},\"type\":\"ConnectorPlacement.EquallySpacedRectSide\",\"uuid\":\"d3309230-0110-441f-b944-3d5d4312a42e\"},{\"content\":{\"connectorIds\":[\"In6\"],\"side\":\"TOP\"},\"type\":\"ConnectorPlacement.EquallySpacedRectSide\",\"uuid\":\"012603a1-4678-4ae1-91f6-3e17a1c8130b\"}]},\"type\":\"ConnectorPlacement.EquallySpacedConnector\",\"uuid\":\"299866d5-057c-44fe-b725-733ff7b8fc12\"}],\"packageUris\":[\"http://schema.mathworks.com/mf0/Connector/19700101\"],\"version\":\"1.0\"}"
  iqd+-ref : Outport
  m : Outport  Port=2
  wires:
  Outer-loop/4(id-*) -> Inner-loop/4(id-*)
  Outer-loop/3(iq-*) -> Inner-loop/3(iq-*)
  Outer-loop/2(id+*) -> Inner-loop/2(id+*)
  Outer-loop/1(iq+*) -> Inner-loop/1(iq+*)
  Block/1 -> Outer-loop/6(Blk)
  vqd+-/1 -> Outer-loop/3(vqd+-)
  freq/1 -> Outer-loop/5(freq)
  iqd+-/1 -> Outer-loop/4(iqd+-)
  Inner-loop/2(id+ref) -> Mux/2
  Pset/1 -> Outer-loop/1(Pset)
  Outer-loop/5(m) -> m/1
  Qset/1 -> Outer-loop/2(Qset)
  Mux/1 -> iqd+-ref/1
  Inner-loop/3(iq-ref) -> Mux/3
  Inner-loop/1(iq+ref) -> Mux/1
  Inner-loop/4(id-ref) -> Mux/4

== system Scenario_3/G1/VSC/VSC Control/Control loops/Phasor I ref ==
  Pset : Inport
  Qset : Inport  Port=2
  vqd+- : Inport  Port=3
  iqd+- : Inport  Port=4
  freq : Inport  Port=5
  Block : Inport  Port=6
  Mux : Mux
  Outer-loop : Subsystem
      settings: PortSchema="{\"entries\":[{\"content\":{\"sides\":[{\"content\":{\"connectorIds\":[\"In1\",\"In2\",\"In3\",\"In4\",\"In5\"]},\"type\":\"ConnectorPlacement.EquallySpacedRectSide\",\"uuid\":\"9a334ab0-c6a2-41fb-a6ec-750715335523\"},{\"content\":{\"connectorIds\":[\"Out1\",\"Out2\",\"Out3\",\"Out4\",\"Out5\"],\"side\":\"RIGHT\"},\"type\":\"ConnectorPlacement.EquallySpacedRectSide\",\"uuid\":\"d3309230-0110-441f-b944-3d5d4312a42e\"},{\"content\":{\"connectorIds\":[\"In6\"],\"side\":\"TOP\"},\"type\":\"ConnectorPlacement.EquallySpacedRectSide\",\"uuid\":\"012603a1-4678-4ae1-91f6-3e17a1c8130b\"}]},\"type\":\"ConnectorPlacement.EquallySpacedConnector\",\"uuid\":\"299866d5-057c-44fe-b725-733ff7b8fc12\"}],\"packageUris\":[\"http://schema.mathworks.com/mf0/Connector/19700101\"],\"version\":\"1.0\"}"
  iqd+-ref : Outport
  m : Outport  Port=2
  wires:
  Outer-loop/4(id-*) -> Mux/4
  Outer-loop/1(iq+*) -> Mux/1
  Outer-loop/3(iq-*) -> Mux/3
  Mux/1 -> iqd+-ref/1
  Qset/1 -> Outer-loop/2(Qset)
  Outer-loop/5(m) -> m/1
  Pset/1 -> Outer-loop/1(Pset)
  Outer-loop/2(id+*) -> Mux/2
  iqd+-/1 -> Outer-loop/4(iqd+-)
  freq/1 -> Outer-loop/5(freq)
  vqd+-/1 -> Outer-loop/3(vqd+-)
  Block/1 -> Outer-loop/6(Blk)

== system Scenario_3/G1/VSC/VSC Control/Control loops/Phasor PQ 1st ==
  Pset : Inport
  Qset : Inport  Port=2
  vqd+- : Inport  Port=3
  iqd+- : Inport  Port=4
  freq : Inport  Port=5
  Block : Inport  Port=6
  Mux : Mux
  Outer-loop : Subsystem
      settings: PortSchema="{\"entries\":[{\"content\":{\"sides\":[{\"content\":{\"connectorIds\":[\"In1\",\"In2\",\"In3\",\"In4\",\"In5\"]},\"type\":\"ConnectorPlacement.EquallySpacedRectSide\",\"uuid\":\"9a334ab0-c6a2-41fb-a6ec-750715335523\"},{\"content\":{\"connectorIds\":[\"Out1\",\"Out2\",\"Out3\",\"Out4\",\"Out5\"],\"side\":\"RIGHT\"},\"type\":\"ConnectorPlacement.EquallySpacedRectSide\",\"uuid\":\"d3309230-0110-441f-b944-3d5d4312a42e\"},{\"content\":{\"connectorIds\":[\"In6\"],\"side\":\"TOP\"},\"type\":\"ConnectorPlacement.EquallySpacedRectSide\",\"uuid\":\"012603a1-4678-4ae1-91f6-3e17a1c8130b\"}]},\"type\":\"ConnectorPlacement.EquallySpacedConnector\",\"uuid\":\"299866d5-057c-44fe-b725-733ff7b8fc12\"}],\"packageUris\":[\"http://schema.mathworks.com/mf0/Connector/19700101\"],\"version\":\"1.0\"}"
  iqd+-ref : Outport
  m : Outport  Port=2
  wires:
  Block/1 -> Outer-loop/6(Blk)
  vqd+-/1 -> Outer-loop/3(vqd+-)
  freq/1 -> Outer-loop/5(freq)
  iqd+-/1 -> Outer-loop/4(iqd+-)
  Outer-loop/2(id+*) -> Mux/2
  Pset/1 -> Outer-loop/1(Pset)
  Outer-loop/5(m) -> m/1
  Qset/1 -> Outer-loop/2(Qset)
  Mux/1 -> iqd+-ref/1
  Outer-loop/3(iq-*) -> Mux/3
  Outer-loop/1(iq+*) -> Mux/1
  Outer-loop/4(id-*) -> Mux/4

== system Scenario_3/G1/VSC/VSC Control/Control loops/SW, EMT AVG, Phasor Quasi-EMT ==
  Pset : Inport
  Qset : Inport  Port=2
  vqd+- : Inport  Port=3
  iqd+- : Inport  Port=4
  freq : Inport  Port=5
  Block : Inport  Port=6
  Inner-loop : Subsystem
      settings: PortSchema="{\"entries\":[{\"content\":{\"sides\":[{\"content\":{\"connectorIds\":[\"In1\",\"In2\",\"In3\",\"In4\"]},\"type\":\"ConnectorPlacement.EquallySpacedRectSide\",\"uuid\":\"8a2e5096-891c-4956-8b6b-4b283c05b7bc\"},{\"content\":{\"connectorIds\":[\"Out1\",\"Out2\",\"Out3\",\"Out4\"],\"side\":\"RIGHT\"},\"type\":\"ConnectorPlacement.EquallySpacedRectSide\",\"uuid\":\"b7af4d2f-ce3f-4dc6-8323-535c80ee1784\"},{\"content\":{\"connectorIds\":[\"In5\",\"In6\",\"In7\"],\"side\":\"TOP\"},\"type\":\"ConnectorPlacement.EquallySpacedRectSide\",\"uuid\":\"1131cb27-465f-45b8-a6a1-03893285239a\"},{\"content\":{\"connectorIds\":[],\"side\":\"BOTTOM\"},\"type\":\"ConnectorPlacement.EquallySpacedRectSide\",\"uuid\":\"c84e74f4-9dae-42a7-97b7-61f404019883\"}]},\"type\":\"ConnectorPlacement.EquallySpacedConnector\",\"uuid\":\"8a900364-1293-46a0-8824-7b0f85f5a81c\"}],\"packageUris\":[\"http://schema.mathworks.com/mf0/Connector/19700101\"],\"version\":\"1.0\"}"
  Mux : Mux
  Outer-loop : Subsystem
      settings: PortSchema="{\"entries\":[{\"content\":{\"sides\":[{\"content\":{\"connectorIds\":[\"In1\",\"In2\",\"In3\",\"In4\",\"In5\"]},\"type\":\"ConnectorPlacement.EquallySpacedRectSide\",\"uuid\":\"9a334ab0-c6a2-41fb-a6ec-750715335523\"},{\"content\":{\"connectorIds\":[\"Out1\",\"Out2\",\"Out3\",\"Out4\",\"Out5\"],\"side\":\"RIGHT\"},\"type\":\"ConnectorPlacement.EquallySpacedRectSide\",\"uuid\":\"d3309230-0110-441f-b944-3d5d4312a42e\"},{\"content\":{\"connectorIds\":[\"In6\"],\"side\":\"TOP\"},\"type\":\"ConnectorPlacement.EquallySpacedRectSide\",\"uuid\":\"012603a1-4678-4ae1-91f6-3e17a1c8130b\"}]},\"type\":\"ConnectorPlacement.EquallySpacedConnector\",\"uuid\":\"299866d5-057c-44fe-b725-733ff7b8fc12\"}],\"packageUris\":[\"http://schema.mathworks.com/mf0/Connector/19700101\"],\"version\":\"1.0\"}"
  vqd+-ref : Outport
  m : Outport  Port=2
  wires:
  Mux/1 -> vqd+-ref/1
  Inner-loop/4(vd-*) -> Mux/4
  Inner-loop/3(vq-*) -> Mux/3
  Inner-loop/2(vd+*) -> Mux/2
  Inner-loop/1(vq+*) -> Mux/1
  Outer-loop/4(id-*) -> Inner-loop/4(id-*)
  Pset/1 -> Outer-loop/1(Pset)
  Qset/1 -> Outer-loop/2(Qset)
  Outer-loop/5(m) -> m/1
  Outer-loop/3(iq-*) -> Inner-loop/3(iq-*)
  freq/1 -> Outer-loop/5(freq)
  iqd+-/1 -> Inner-loop/7(iqd+-), Outer-loop/4(iqd+-)
  Block/1 -> Inner-loop/5(Blk), Outer-loop/6(Blk)
  vqd+-/1 -> Inner-loop/6(vqd+-), Outer-loop/3(vqd+-)
  Outer-loop/2(id+*) -> Inner-loop/2(id+*)
  Outer-loop/1(iq+*) -> Inner-loop/1(iq+*)
